simulink model "mass_spring_damper_AMPC_with_RLS"  (R2019b)
settings: Solver=VariableStepAuto  StartTime=0.0  StopTime=100  FixedStep=0.01  RelTol=1e-3
values from neighbouring files (symbols this model uses):
  A = AB(:,1:2)    [DMDc_MW.m]    (also in DMDc_param_sweep.m = real(A); EKF_msd_estimator.m = [0, 1; -k/m, -b/m]; HAVOK.m = AB(:,1:q*m); HAVOK_param_sweep.m = real(A))
  B = AB(:,end)    [DMDc_MW.m]    (also in DMDc_param_sweep.m = AB(:,(q*m+1):end); EKF_estimator.m = zeros(nx,1); EKF_msd_estimator.m = [0; 1/m]; HAVOK.m = AB(:,(q*m+1):end))
  C = [0 1]    [DMDc_MW.m]    (also in EKF_estimator.m = eye(6); EKF_msd_estimator.m = [1, 0]; KF_estimator.m = [1, 0]; LS.m)
  D = 0    [DMDc_MW.m]    (also in DMDc_param_sweep.m = (q-1)*Ts; EKF_estimator.m = m*L*L*(M+m*(1-Cx^2)); EKF_msd_estimator.m; HAVOK.m = 3.99)
  DX = [0; 0]    [DMDc_MW.m]    (also in LS.m; cart_pend_DMD_script.m; convert_model_for_AMPC.m; mass_spring_damper_DMD_script.m)
  nu = size_B(2)    [DMDc_MW.m]    (also in EKF_msd_estimator.m = 1; LS.m; Linear_regression_state_estimator.m = 2; cart_pend_DMD_script.m)
  ny = size_C(1)    [DMDc_MW.m]    (also in EKF_msd_estimator.m = 1; LS.m; Linear_regression_state_estimator.m = 1; cart_pend_DMD_script.m)
  p = 200    [HAVOK.m]    (also in cart_pend_HAVOK_N_train_time_sweep.m = p_saved(index); cart_pend_HAVOK_script.m = 40; floating_pend_2D_HAVOK_script.m = p_saved(save_index); mass_spring_damper_DMD_script.m = size(V)*[0; 1])
  U = zeros(nu,1)    [DMDc_MW.m]    (also in HAVOK.m = u_train(:, q:end-1); LS.m; Linear_regression_state_estimator.m = reshape(U, nx*nu,1); cart_pend_DMD_script.m)
  X = zeros(nx,1)    [DMDc_MW.m]    (also in LS.m; Linear_regression_parameter_estimator.m = [y_data(2:end-1)', y_data(1:end-2)', u_data(1:end-2)']; cart_pend_DMD_script.m; cart_pend_HAVOK_N_train_error_sweep.m = zeros(q*m,w))
  Y = zeros(ny,1)    [DMDc_MW.m]    (also in DMDc_param_sweep.m = zeros(q*m,w); HAVOK.m = zeros(q*m,w); HAVOK_param_sweep.m = zeros(q*m,w); LS.m)
undefined symbols (not defined in the file or in its folder): blk, iA, isLTV, lastPcov, lastu, lastx, MDscale, MVscale, nCC, nud, nv, nxp, nym, RMVscale, RYscale, ts, uoff, xoff, Yscale
libraries: mpcsigdimcheck_private x23
(part 1 of 2)
settings Model: Creator=Murray  LastModifiedBy=Murray

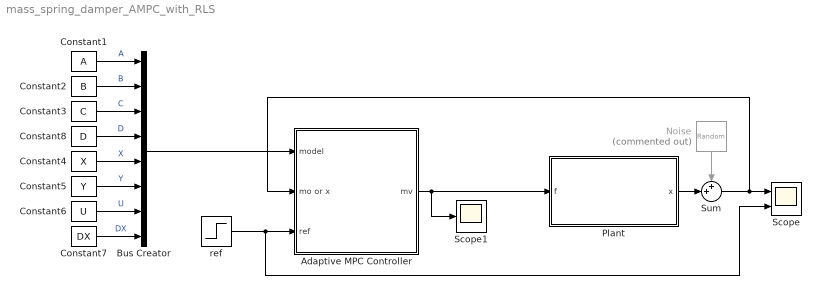
== system mass_spring_damper_AMPC_with_RLS ==
  Adaptive MPC Controller : Subsystem  AncestorBlock=mpclib/Adaptive MPC Controller  SCDEnableBlockLinearizationSpecification=on  InitFcn=ampcblock_InitFcn  StartFcn=ampcblock_StartFcn  mask(Adaptive MPC){mpcobj=mpc1, x0=, enable_value=0, updateMPCinCallerWorkspace=on, md_inport=off, mv_inport=off, uref_inport=off, return_cost=off, return_mvseq=off, return_qpstatus=off, return_xseq=off, return_state=off, return_ovseq=off, state_inport=off, isltv_plant=off, umin_inport=off, umax_inport=off, ymin_inport=off, ymax_inport=off, cc_inport=off, ywt_inport=off, uwt_inport=off, duwt_inport=off, rhoeps_inport=off, pm_inport=off, MaximumP=10, HorizonChoice=FixedHorizon, BlockDataType=double, SampleTimeInherited=off, switch_inport=off}
      mask prompts: mpcobj "MPC:general:BlgAMPC"; x0 "MPC:general:BlgState"; enable_value "Value enabling optimization"; updateMPCinCallerWorkspace "Update MPC object in caller workspace"; md_inport "MPC:general:BlgMD"; mv_inport "MPC:general:BlgEXTMV"; uref_inport "MPC:general:BlgMVTARGET"; return_cost "MPC:general:BlgCOST"; return_mvseq "MPC:general:BlgMVSEQ"; return_qpstatus "MPC:general:BlgQPSTATUS"; return_xseq "MPC:general:BlgXSEQ"; return_state "MPC:general:BlgESTSTATE"; return_ovseq "MPC:general:BlgOVSEQ"; state_inport "MPC:general:BlgXKK"; isltv_plant "MPC:general:BlgLTV"; umin_inport "MPC:general:BlgMVMin"; umax_inport "MPC:general:BlgMVMax"; ymin_inport "MPC:general:BlgOVMin"; ymax_inport "MPC:general:BlgOVMax"; cc_inport "Custom constraints (E, F, G, S)"; ywt_inport "MPC:general:BlgYWT"; uwt_inport "MPC:general:BlgUWT"; duwt_inport "MPC:general:BlgDUWT"; rhoeps_inport "MPC:general:BlgECRWT"; pm_inport "MPC:general:BlgPM"; MaximumP "MPC:general:BlgMaximumP"; HorizonChoice "Simulink:Variants:LabelComboBox"; BlockDataType "MPC:general:BlgDATATYPE"; SampleTimeInherited "MPC:general:BlgTS"; switch_inport "MPC:general:BlgSWITCH"
      mask help: MPC:utility:MaskDescAdaptiveMPC1
      mask init:
      | [blk,ts,A,B,C,D,isQP,strmoorx,nmoorx,nu,nv,ny,nx,nym,nud,...
      |     degrees,lastPcov,H,Hinv,Linv,iA,Ac,Kx,Ku1,Kut,Kr,Kv,...
      |     Mlim,Mx,Mu1,Mv,z_degrees,utarget,...
      |     lastx,lastu,p,xoff,uoff,yoff,voff,myoff,no_md,no_ref,...
      |     maxiter,CustomSolver,CustomSolverCodeGen,UseWarmStart,UseSuboptimalSolution,...
      |     nxQP,openloopflag,no_ym,no_mv,no_uref,...
      |     no_umin,no_umax,no_ymin,no_ymax,no_cc,...
      |     no_switch,CustomEstimation,...
      |     no_ywt, no_uwt, no_duwt, no_rhoeps,...
      |     Wy,Wdu,Jm,SuJm,Su1,Sx,Hv,Wu,I1,...
      |     isAdaptive, isLTV, Mrows, nCC, Ecc, Fcc, Scc, Gcc, Cid, Did, ...
      |     nxp, nup, nxid, mvindex, mdindex, unindex, myindex, ...
      |     Uscale, Yscale, MVscale, MDscale, ...
      |     RYscale,RMYscale,RMVscale,RMDscale,no_p,no_m,p0] = ampcblock_MaskInitFcnParameter();
      | ampcblock_MaskInitFcnResize(gcb,nv,nu,ny,nCC);
      mask Help: eval('mpcCSHelp(''MPCmaskAdaptive'',''HelpBrowser'')');
      mask Callback pm_inport: mpcblocks_callbackPM(gcb);
      mask TypeOptions HorizonChoice: MPC/optimizer/LabelModeActiveChoice
      mask DialogControl mpcobj Prompt: Adaptive MPC Controller
      mask DialogControl x0 Prompt: Initial Controller State
      mask DialogControl Container5 Prompt: MPC:general:BlgTab1
      mask DialogControl Container6 Prompt: MPC:general:BlgBox11
      mask DialogControl md_inport Prompt: Measured disturbance (md)
      mask DialogControl mv_inport Prompt: External manipulated variable (ext.mv)
      mask DialogControl uref_inport Prompt: Targets for manipulated variables (mv.target)
      mask DialogControl Container7 Prompt: MPC:general:BlgBox12
      mask DialogControl return_cost Prompt: Optimal cost (cost)
      mask DialogControl return_mvseq Prompt: Optimal control sequence (mv.seq)
      mask DialogControl return_qpstatus Prompt: Optimization status (qp.status)
      mask DialogControl return_xseq Prompt: Optimal state sequence (x.seq)
      mask DialogControl return_state Prompt: Estimated controller states (est.state)
      mask DialogControl return_ovseq Prompt: Optimal output sequence (y.seq)
      mask DialogControl Container16 Prompt: MPC:general:BlgBox13
      mask DialogControl state_inport Prompt: Use custom state estimation instead of using the built-in Kalman filter (x[k|k])
      mask DialogControl Container9 Prompt: MPC:general:BlgTab2
      mask DialogControl Container19 Prompt: MPC:general:BlgBox20
      mask DialogControl isltv_plant Prompt: Linear Time-Varying (LTV) plants (model expects 3-D signals)
      mask DialogControl Container10 Prompt: MPC:general:BlgBox21
      mask DialogControl umin_inport Prompt: Lower MV limits (umin)
      mask DialogControl umax_inport Prompt: Upper MV limits (umax)
      mask DialogControl ymin_inport Prompt: Lower OV limits (ymin)
      mask DialogControl ymax_inport Prompt: Upper OV limits (ymax)
      mask DialogControl Container11 Prompt: MPC:general:BlgBox22
      mask DialogControl ywt_inport Prompt: OV weights (y.wt)
      mask DialogControl uwt_inport Prompt: MV weights (u.wt)
      mask DialogControl duwt_inport Prompt: MVRate weights (du.wt)
      mask DialogControl rhoeps_inport Prompt: Slack variable weight (ecr.wt)
      mask DialogControl Container17 Prompt: Prediction and Control Horizons
      mask DialogControl pm_inport Prompt: Adjust prediction horizon (p) and control horizon (m) at run time
      mask DialogControl MaximumP Prompt: Maximum prediction horizon
      mask DialogControl HorizonChoice Prompt: Label mode active choice:
      mask DialogControl Container13 Prompt: MPC:general:BlgTab3
      mask DialogControl Container14 Prompt: MPC:general:BlgBox31
      mask DialogControl BlockDataType Prompt: Block Data Type
      mask DialogControl Container15 Prompt: MPC:general:BlgBox32
      mask DialogControl SampleTimeInherited Prompt: Inherit sample time (must be the same as controller sample time)
      mask DialogControl Container18 Prompt: MPC:general:BlgBox33
      mask DialogControl switch_inport Prompt: Use external signal to enable or disable optimization (switch)
      mask Display:
      | fprintf('Adaptive\nMPC');
      | port_label('output', 1, 'mv')
      | port_label('input', 1, 'model')
      | port_label('input', 2, 'mo')
      | port_label('input', 3, 'ref')
  Bus Creator : BusCreator  Inputs=A,B,C,D,X,Y,U,DX
  Constant1 : Constant  Value=A
  Constant2 : Constant  Value=B
  Constant3 : Constant  Value=C
  Constant4 : Constant  Value=X
  Constant5 : Constant  Value=Y
  Constant6 : Constant  Value=U
  Constant7 : Constant  Value=DX
  Constant8 : Constant  Value=D
  Noise : RandomNumber  Commented=on  Variance=0.00001  SampleTime=0.01
  Plant : Subsystem
  Scope : Scope  NumInputPorts=2
  Scope1 : Scope
  Sum : Sum  Inputs=++|
  ref : Step  SampleTime=0
  wires:
  ref/1 -> Adaptive MPC Controller/3(ref), Scope/2
  Adaptive MPC Controller/1(mv) -> Scope1/1, Plant/1(f)
  Constant1/1 -> Bus Creator/1  "A"
  Constant2/1 -> Bus Creator/2  "B"
  Constant6/1 -> Bus Creator/7  "U"
  Constant5/1 -> Bus Creator/6  "Y"
  Constant4/1 -> Bus Creator/5  "X"
  Constant8/1 -> Bus Creator/4  "D"
  Constant3/1 -> Bus Creator/3  "C"
  Bus Creator/1 -> Adaptive MPC Controller/1(model)
  Constant7/1 -> Bus Creator/8  "DX"
  Noise/1 -> Sum/1
  Plant/1(x) -> Sum/2
  Sum/1 -> Adaptive MPC Controller/2(mo or x), Scope/1

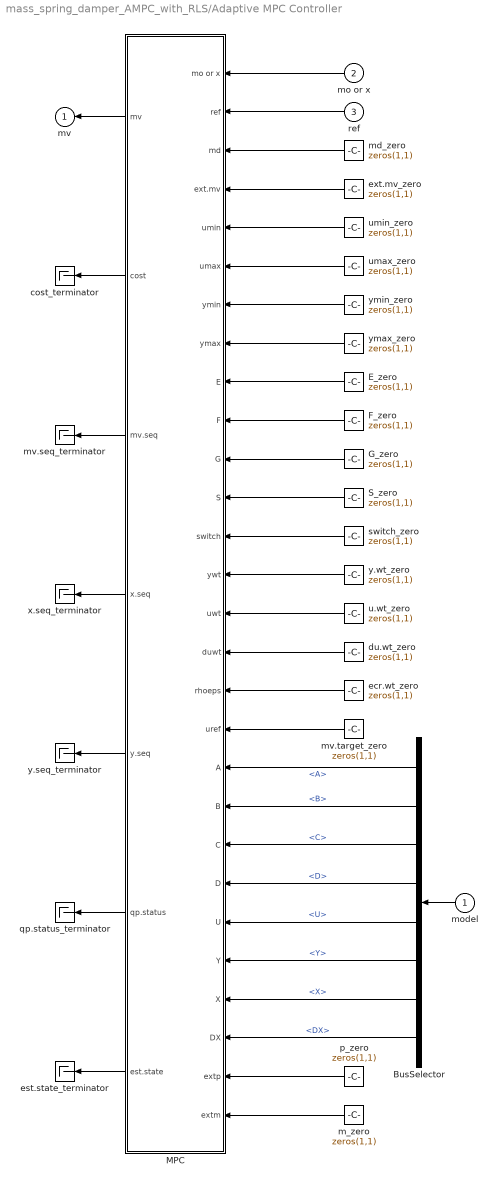
== system mass_spring_damper_AMPC_with_RLS/Adaptive MPC Controller ==
  model : Inport
  mo or x : Inport  Port=2
  ref : Inport  Port=3
  BusSelector : BusSelector  OutputSignals=A,B,C,D,U,Y,X,DX
  E_zero : Constant  Value=zeros(1,1)  VectorParams1D=off  OutDataTypeStr=BlockDataType
  F_zero : Constant  Value=zeros(1,1)  VectorParams1D=off  OutDataTypeStr=BlockDataType
  G_zero : Constant  Value=zeros(1,1)  VectorParams1D=off  OutDataTypeStr=BlockDataType
  MPC : Subsystem
  S_zero : Constant  Value=zeros(1,1)  VectorParams1D=off  OutDataTypeStr=BlockDataType
  cost_terminator : Terminator
  du.wt_zero : Constant  Value=zeros(1,1)  OutDataTypeStr=BlockDataType
  ecr.wt_zero : Constant  Value=zeros(1,1)  OutDataTypeStr=BlockDataType
  est.state_terminator : Terminator
  ext.mv_zero : Constant  Value=zeros(1,1)  OutDataTypeStr=BlockDataType
  m_zero : Constant  Value=zeros(1,1)  OutDataTypeStr=BlockDataType
  md_zero : Constant  Value=zeros(1,1)  OutDataTypeStr=BlockDataType
  mv.seq_terminator : Terminator
  mv.target_zero : Constant  Value=zeros(1,1)  OutDataTypeStr=BlockDataType
  p_zero : Constant  Value=zeros(1,1)  OutDataTypeStr=BlockDataType
  qp.status_terminator : Terminator
  switch_zero : Constant  Value=zeros(1,1)  OutDataTypeStr=BlockDataType
  u.wt_zero : Constant  Value=zeros(1,1)  OutDataTypeStr=BlockDataType
  umax_zero : Constant  Value=zeros(1,1)  OutDataTypeStr=BlockDataType
  umin_zero : Constant  Value=zeros(1,1)  OutDataTypeStr=BlockDataType
  x.seq_terminator : Terminator
  y.seq_terminator : Terminator
  y.wt_zero : Constant  Value=zeros(1,1)  OutDataTypeStr=BlockDataType
  ymax_zero : Constant  Value=zeros(1,1)  OutDataTypeStr=BlockDataType
  ymin_zero : Constant  Value=zeros(1,1)  OutDataTypeStr=BlockDataType
  mv : Outport  VectorParamsAs1DForOutWhenUnconnected=off
  wires:
  m_zero/1 -> MPC/28(extm)
  p_zero/1 -> MPC/27(extp)
  MPC/5(y.seq) -> y.seq_terminator/1
  MPC/4(x.seq) -> x.seq_terminator/1
  G_zero/1 -> MPC/11(G)
  F_zero/1 -> MPC/10(F)
  E_zero/1 -> MPC/9(E)
  S_zero/1 -> MPC/12(S)
  MPC/7(est.state) -> est.state_terminator/1
  y.wt_zero/1 -> MPC/14(ywt)
  switch_zero/1 -> MPC/13(switch)
  ymin_zero/1 -> MPC/7(ymin)
  umax_zero/1 -> MPC/6(umax)
  umin_zero/1 -> MPC/5(umin)
  u.wt_zero/1 -> MPC/15(uwt)
  ymax_zero/1 -> MPC/8(ymax)
  du.wt_zero/1 -> MPC/16(duwt)
  ecr.wt_zero/1 -> MPC/17(rhoeps)
  mv.target_zero/1 -> MPC/18(uref)
  ext.mv_zero/1 -> MPC/4(ext.mv)
  BusSelector/8 -> MPC/26(DX)  "<DX>"
  BusSelector/7 -> MPC/25(X)  "<X>"
  BusSelector/6 -> MPC/24(Y)  "<Y>"
  BusSelector/5 -> MPC/23(U)  "<U>"
  model/1 -> BusSelector/1
  BusSelector/4 -> MPC/22(D)  "<D>"
  BusSelector/3 -> MPC/21(C)  "<C>"
  BusSelector/2 -> MPC/20(B)  "<B>"
  BusSelector/1 -> MPC/19(A)  "<A>"
  MPC/6(qp.status) -> qp.status_terminator/1
  MPC/3(mv.seq) -> mv.seq_terminator/1
  MPC/2(cost) -> cost_terminator/1
  ref/1 -> MPC/2(ref)
  mo or x/1 -> MPC/1(mo or x)
  MPC/1(mv) -> mv/1
  md_zero/1 -> MPC/3(md)

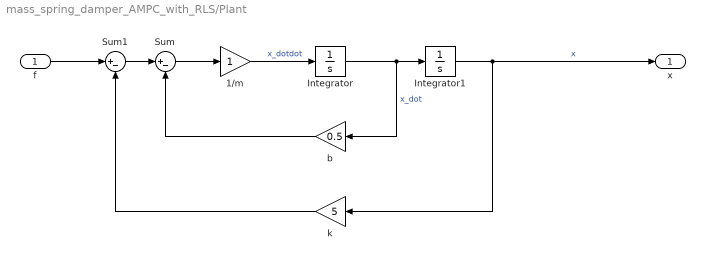
== system mass_spring_damper_AMPC_with_RLS/Plant ==
  f : Inport
  1/m : Gain
  Integrator : Integrator
  Integrator1 : Integrator
  Sum : Sum  Inputs=|+-
  Sum1 : Sum  Inputs=|+-
  b : Gain  Gain=0.5
  k : Gain  Gain=5
  x : Outport
  wires:
  f/1 -> Sum1/1
  Integrator/1 -> b/1, Integrator1/1  "x_dot"
  Sum1/1 -> Sum/1
  1/m/1 -> Integrator/1  "x_dotdot"
  Integrator1/1 -> x/1, k/1  "x"
  Sum/1 -> 1/m/1
  b/1 -> Sum/2
  k/1 -> Sum1/2

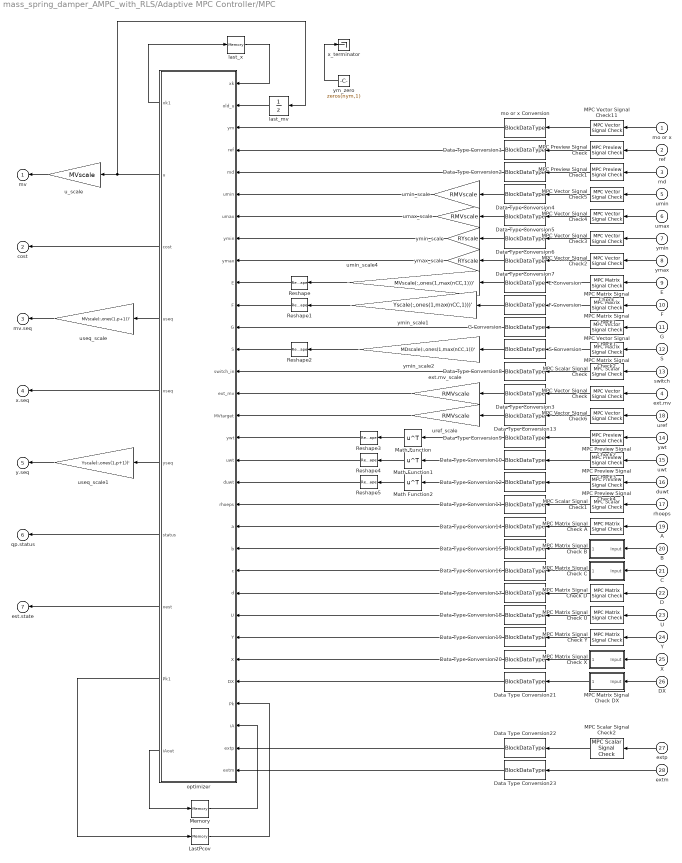
== system mass_spring_damper_AMPC_with_RLS/Adaptive MPC Controller/MPC ==
  mo or x : Inport
  ref : Inport  Port=2
  md : Inport  Port=3
  ext.mv : Inport  Port=4
  umin : Inport  Port=5
  umax : Inport  Port=6
  ymin : Inport  Port=7
  ymax : Inport  Port=8
  E : Inport  Port=9
  F : Inport  Port=10
  G : Inport  Port=11
  S : Inport  Port=12
  switch : Inport  Port=13
  ywt : Inport  Port=14
  uwt : Inport  Port=15
  duwt : Inport  Port=16
  rhoeps : Inport  Port=17
  uref : Inport  Port=18
  A : Inport  Port=19
  B : Inport  Port=20
  C : Inport  Port=21
  D : Inport  Port=22
  U : Inport  Port=23
  Y : Inport  Port=24
  X : Inport  Port=25
  DX : Inport  Port=26
  extp : Inport  Port=27
  extm : Inport  Port=28
  Data Type Conversion{1..23} (23 alike) : DataTypeConversion  OutDataTypeStr=BlockDataType
  E Conversion : DataTypeConversion  OutDataTypeStr=BlockDataType
  F Conversion : DataTypeConversion  OutDataTypeStr=BlockDataType
  G Conversion : DataTypeConversion  OutDataTypeStr=BlockDataType
  LastPcov : Memory  InitialCondition=lastPcov  InheritSampleTime=on  LinearizeAsDelay=on
  MPC Matrix Signal Check : mpcsigdimcheck_private/MPC Matrix Signal Check  blockname=blk  signalname='CustomConstraint.E'  numrow=max(nCC,1)  numcol=nu  steps=0  isLTV=0
      settings: SourceProductName=Model Predictive Control Toolbox  SourceProductBaseCode=MP
  MPC Matrix Signal Check A : mpcsigdimcheck_private/MPC Matrix Signal Check  blockname=blk  signalname='Model.A'  numrow=nxp  numcol=nxp  steps=p  isLTV=isLTV
      settings: SourceProductName=Model Predictive Control Toolbox  SourceProductBaseCode=MP
  MPC Matrix Signal Check B : Subsystem  AncestorBlock=mpcsigdimcheck_private/MPC Matrix Signal Check  mask(MPCSignalDimensionCheck){blockname=blk, signalname='Model.B', numrow=nxp, numcol=nu+nv-1+nud, steps=p, isLTV=isLTV}
      mask prompts: blockname "Block name"; signalname "Signal name"; numrow "Number of rows"; numcol "Number of columns"; steps "Number of prediction steps"; isLTV "Linear Time-Varying (LTV) plants"
      mask help: Internal use to check MPC input signal dimensions at compile time.
      mask init:
      | nrow = uint16(numrow);
      | ncol = uint16(numcol);
      | nsteps = uint16(steps);
      | isltv = uint16(isLTV);
  MPC Matrix Signal Check C : Subsystem  AncestorBlock=mpcsigdimcheck_private/MPC Matrix Signal Check  mask(MPCSignalDimensionCheck){blockname=blk, signalname='Model.C', numrow=ny, numcol=nxp, steps=p, isLTV=isLTV}
      mask prompts: blockname "Block name"; signalname "Signal name"; numrow "Number of rows"; numcol "Number of columns"; steps "Number of prediction steps"; isLTV "Linear Time-Varying (LTV) plants"
      mask help: Internal use to check MPC input signal dimensions at compile time.
      mask init:
      | nrow = uint16(numrow);
      | ncol = uint16(numcol);
      | nsteps = uint16(steps);
      | isltv = uint16(isLTV);
  MPC Matrix Signal Check D : mpcsigdimcheck_private/MPC Matrix Signal Check  blockname=blk  signalname='Model.D'  numrow=ny  numcol=nu+nv-1+nud  steps=p  isLTV=isLTV
      settings: SourceProductName=Model Predictive Control Toolbox  SourceProductBaseCode=MP
  MPC Matrix Signal Check DX : Subsystem  AncestorBlock=mpcsigdimcheck_private/MPC Matrix Signal Check  mask(MPCSignalDimensionCheck){blockname=blk, signalname='Model.DX', numrow=nxp, numcol=1, steps=p, isLTV=isLTV}
      mask prompts: blockname "Block name"; signalname "Signal name"; numrow "Number of rows"; numcol "Number of columns"; steps "Number of prediction steps"; isLTV "Linear Time-Varying (LTV) plants"
      mask help: Internal use to check MPC input signal dimensions at compile time.
      mask init:
      | nrow = uint16(numrow);
      | ncol = uint16(numcol);
      | nsteps = uint16(steps);
      | isltv = uint16(isLTV);
  MPC Matrix Signal Check U : mpcsigdimcheck_private/MPC Matrix Signal Check  blockname=blk  signalname='Model.U'  numrow=nu+nv-1+nud  numcol=1  steps=p  isLTV=isLTV
      settings: SourceProductName=Model Predictive Control Toolbox  SourceProductBaseCode=MP
  MPC Matrix Signal Check X : Subsystem  AncestorBlock=mpcsigdimcheck_private/MPC Matrix Signal Check  mask(MPCSignalDimensionCheck){blockname=blk, signalname='Model.X', numrow=nxp, numcol=1, steps=p, isLTV=isLTV}
      mask prompts: blockname "Block name"; signalname "Signal name"; numrow "Number of rows"; numcol "Number of columns"; steps "Number of prediction steps"; isLTV "Linear Time-Varying (LTV) plants"
      mask help: Internal use to check MPC input signal dimensions at compile time.
      mask init:
      | nrow = uint16(numrow);
      | ncol = uint16(numcol);
      | nsteps = uint16(steps);
      | isltv = uint16(isLTV);
  MPC Matrix Signal Check Y : mpcsigdimcheck_private/MPC Matrix Signal Check  blockname=blk  signalname='Model.Y'  numrow=ny  numcol=1  steps=p  isLTV=isLTV
      settings: SourceProductName=Model Predictive Control Toolbox  SourceProductBaseCode=MP
  MPC Matrix Signal Check1 : mpcsigdimcheck_private/MPC Matrix Signal Check  blockname=blk  signalname='CustomConstraint.F'  numrow=max(nCC,1)  numcol=ny  steps=0  isLTV=0
      settings: SourceProductName=Model Predictive Control Toolbox  SourceProductBaseCode=MP
  MPC Matrix Signal Check2 : mpcsigdimcheck_private/MPC Matrix Signal Check  blockname=blk  signalname='CustomConstraint.S'  numrow=max(nCC,1)  numcol=max(nv-1,1)  steps=0  isLTV=0
      settings: SourceProductName=Model Predictive Control Toolbox  SourceProductBaseCode=MP
  MPC Preview Signal Check : mpcsigdimcheck_private/MPC Preview Signal Check  blockname=blk  signalname='ref'  numrow=p  numcol=ny
      settings: SourceProductName=Model Predictive Control Toolbox  SourceProductBaseCode=MP
  MPC Preview Signal Check1 : mpcsigdimcheck_private/MPC Preview Signal Check  blockname=blk  signalname='md'  numrow=p+1  numcol=max(nv-1,1)
      settings: SourceProductName=Model Predictive Control Toolbox  SourceProductBaseCode=MP
  MPC Preview Signal Check2 : mpcsigdimcheck_private/MPC Preview Signal Check  blockname=blk  signalname='y.wt'  numrow=p  numcol=ny
      settings: SourceProductName=Model Predictive Control Toolbox  SourceProductBaseCode=MP
  MPC Preview Signal Check3 : mpcsigdimcheck_private/MPC Preview Signal Check  blockname=blk  signalname='u.wt'  numrow=p  numcol=nu
      settings: SourceProductName=Model Predictive Control Toolbox  SourceProductBaseCode=MP
  MPC Preview Signal Check4 : mpcsigdimcheck_private/MPC Preview Signal Check  blockname=blk  signalname='du.wt'  numrow=p  numcol=nu
      settings: SourceProductName=Model Predictive Control Toolbox  SourceProductBaseCode=MP
  MPC Scalar Signal Check : mpcsigdimcheck_private/MPC Scalar Signal Check  blockname=blk  signalname='switch'
      settings: SourceProductName=Model Predictive Control Toolbox  SourceProductBaseCode=MP
  MPC Scalar Signal Check1 : mpcsigdimcheck_private/MPC Scalar Signal Check  blockname=blk  signalname='ecr.wt'
      settings: SourceProductName=Model Predictive Control Toolbox  SourceProductBaseCode=MP
  MPC Scalar Signal Check2 : mpcsigdimcheck_private/MPC Scalar Signal Check  blockname=blk  signalname='p'
      settings: SourceProductName=Model Predictive Control Toolbox  SourceProductBaseCode=MP
  MPC Vector Signal Check : mpcsigdimcheck_private/MPC Vector Signal Check  blockname=blk  signalname='ext.mv'  num=nu  vectortype=Any
      settings: SourceProductName=Model Predictive Control Toolbox  SourceProductBaseCode=MP
  MPC Vector Signal Check1 : mpcsigdimcheck_private/MPC Vector Signal Check  blockname=blk  signalname='CustomConstraint.G'  num=max(nCC,1)  vectortype=Column
      settings: SourceProductName=Model Predictive Control Toolbox  SourceProductBaseCode=MP
  MPC Vector Signal Check11 : mpcsigdimcheck_private/MPC Vector Signal Check  blockname=blk  signalname=strmoorx  num=nmoorx  vectortype=Any
      settings: SourceProductName=Model Predictive Control Toolbox  SourceProductBaseCode=MP
  MPC Vector Signal Check2 : mpcsigdimcheck_private/MPC Vector Signal Check  blockname=blk  signalname='ymax'  num=ny  vectortype=Any
      settings: SourceProductName=Model Predictive Control Toolbox  SourceProductBaseCode=MP
  MPC Vector Signal Check3 : mpcsigdimcheck_private/MPC Vector Signal Check  blockname=blk  signalname='ymin'  num=ny  vectortype=Any
      settings: SourceProductName=Model Predictive Control Toolbox  SourceProductBaseCode=MP
  MPC Vector Signal Check4 : mpcsigdimcheck_private/MPC Vector Signal Check  blockname=blk  signalname='umax'  num=nu  vectortype=Any
      settings: SourceProductName=Model Predictive Control Toolbox  SourceProductBaseCode=MP
  MPC Vector Signal Check5 : mpcsigdimcheck_private/MPC Vector Signal Check  blockname=blk  signalname='umin'  num=nu  vectortype=Any
      settings: SourceProductName=Model Predictive Control Toolbox  SourceProductBaseCode=MP
  MPC Vector Signal Check6 : mpcsigdimcheck_private/MPC Vector Signal Check  blockname=blk  signalname='mv.target'  num=nu  vectortype=Any
      settings: SourceProductName=Model Predictive Control Toolbox  SourceProductBaseCode=MP
  Math Function : Math  Operator=transpose  SaturateOnIntegerOverflow=on
  Math Function1 : Math  Operator=transpose  SaturateOnIntegerOverflow=on
  Math Function2 : Math  Operator=transpose  SaturateOnIntegerOverflow=on
  Memory : Memory  InitialCondition=iA  InheritSampleTime=on  LinearizeAsDelay=on
  Reshape : Reshape  OutputDimensionality=Customize  OutputDimensions=double([max(nCC,1),nu])
  Reshape1 : Reshape  OutputDimensionality=Customize  OutputDimensions=double([max(nCC,1),ny])
  Reshape2 : Reshape  OutputDimensionality=Customize  OutputDimensions=double([max(nCC,1),max(nv-1,1)])
  Reshape3 : Reshape  OutputDimensionality=Column vector (2-D)
  Reshape4 : Reshape  OutputDimensionality=Column vector (2-D)
  Reshape5 : Reshape  OutputDimensionality=Column vector (2-D)
  S Conversion : DataTypeConversion  OutDataTypeStr=BlockDataType
  ext.mv_scale : Gain  Gain=RMVscale  SampleTime=ts
  last_mv : UnitDelay  InitialCondition=lastu+uoff  SampleTime=ts  HasFrameUpgradeWarning=on
  last_x : Memory  InitialCondition=lastx+xoff  InheritSampleTime=on  LinearizeAsDelay=on
  mo or x Conversion : DataTypeConversion  OutDataTypeStr=BlockDataType
  optimizer : Subsystem  VariantControlMode=Label  Variant=on  VariantControl=Variant1  LabelModeActiveChoice=FixedHorizon
  u_scale : Gain  Gain=MVscale  SampleTime=ts
  umax_scale : Gain  Gain=RMVscale  SampleTime=ts
  umin_scale : Gain  Gain=RMVscale  SampleTime=ts
  umin_scale4 : Gain  Gain=MVscale(:,ones(1,max(nCC,1)))'  SampleTime=ts
  uref_scale : Gain  Gain=RMVscale  SampleTime=ts
  useq_scale : Gain  Gain=MVscale(:,ones(1,p+1))'  SampleTime=ts
  useq_scale1 : Gain  Gain=Yscale(:,ones(1,p+1))'  SampleTime=ts
  x_terminator : Terminator
  ym_zero : Constant  Value=zeros(nym,1)  OutDataTypeStr=BlockDataType
  ymax_scale : Gain  Gain=RYscale  SampleTime=ts
  ymin_scale : Gain  Gain=RYscale  SampleTime=ts
  ymin_scale1 : Gain  Gain=Yscale(:,ones(1,max(nCC,1)))'  SampleTime=ts
  ymin_scale2 : Gain  Gain=MDscale(:,ones(1,max(nCC,1)))'  SampleTime=ts
  mv : Outport  OutDataTypeStr=BlockDataType  VectorParamsAs1DForOutWhenUnconnected=off
  cost : Outport  Port=2  OutDataTypeStr=BlockDataType  VectorParamsAs1DForOutWhenUnconnected=off
  mv.seq : Outport  Port=3  OutDataTypeStr=BlockDataType  VectorParamsAs1DForOutWhenUnconnected=off
  x.seq : Outport  Port=4  OutDataTypeStr=BlockDataType  VectorParamsAs1DForOutWhenUnconnected=off
  y.seq : Outport  Port=5  OutDataTypeStr=BlockDataType  VectorParamsAs1DForOutWhenUnconnected=off
  qp.status : Outport  Port=6  OutDataTypeStr=BlockDataType  VectorParamsAs1DForOutWhenUnconnected=off
  est.state : Outport  Port=7  OutDataTypeStr=BlockDataType  VectorParamsAs1DForOutWhenUnconnected=off
  wires:
  MPC Scalar Signal Check2/1 -> Data Type Conversion22/1
  extm/1 -> Data Type Conversion23/1
  extp/1 -> MPC Scalar Signal Check2/1
  Data Type Conversion23/1 -> optimizer/32(extm)
  Data Type Conversion22/1 -> optimizer/31(extp)
  optimizer/10(" iAout") -> Memory/1
  optimizer/9(" Pk1") -> LastPcov/1
  optimizer/8(" xest") -> est.state/1
  optimizer/7(" status") -> qp.status/1
  optimizer/6(" yseq") -> useq_scale1/1
  optimizer/5(" xseq") -> x.seq/1
  optimizer/4(" useq") -> useq_scale/1
  optimizer/3(" cost") -> cost/1
  optimizer/2(" u") -> last_mv/1, u_scale/1
  optimizer/1(" xk1") -> last_x/1
  Memory/1 -> optimizer/30("iA ")
  LastPcov/1 -> optimizer/29("Pk ")
  Data Type Conversion21/1 -> optimizer/28("DX ")
  Data Type Conversion20/1 -> optimizer/27("X ")
  Data Type Conversion19/1 -> optimizer/26("Y ")
  Data Type Conversion18/1 -> optimizer/25("U ")
  Data Type Conversion17/1 -> optimizer/24("d ")
  Data Type Conversion16/1 -> optimizer/23("c ")
  Data Type Conversion15/1 -> optimizer/22("b ")
  Data Type Conversion14/1 -> optimizer/21("a ")
  Data Type Conversion11/1 -> optimizer/20("rhoeps ")
  Reshape5/1 -> optimizer/19("duwt ")
  Reshape4/1 -> optimizer/18("uwt ")
  Reshape3/1 -> optimizer/17("ywt ")
  uref_scale/1 -> optimizer/16("MVtarget ")
  ext.mv_scale/1 -> optimizer/15("ext_mv ")
  Data Type Conversion8/1 -> optimizer/14("switch_in ")
  Reshape2/1 -> optimizer/13("S ")
  G Conversion/1 -> optimizer/12("G ")
  Reshape1/1 -> optimizer/11("F ")
  Reshape/1 -> optimizer/10("E ")
  ymax_scale/1 -> optimizer/9("ymax ")
  ymin_scale/1 -> optimizer/8("ymin ")
  umax_scale/1 -> optimizer/7("umax ")
  umin_scale/1 -> optimizer/6("umin ")
  Data Type Conversion2/1 -> optimizer/5("md ")
  Data Type Conversion1/1 -> optimizer/4("ref ")
  mo or x Conversion/1 -> optimizer/3("ym ")
  last_mv/1 -> optimizer/2("old_u ")
  last_x/1 -> optimizer/1("xk ")
  useq_scale1/1 -> y.seq/1
  Math Function2/1 -> Reshape5/1
  Math Function1/1 -> Reshape4/1
  Math Function/1 -> Reshape3/1
  MPC Matrix Signal Check1/1 -> F Conversion/1
  umin_scale4/1 -> Reshape/1
  ymin_scale1/1 -> Reshape1/1
  G/1 -> MPC Vector Signal Check1/1
  F/1 -> MPC Matrix Signal Check1/1
  E Conversion/1 -> umin_scale4/1
  ymin_scale2/1 -> Reshape2/1
  MPC Matrix Signal Check/1 -> E Conversion/1
  S/1 -> MPC Matrix Signal Check2/1
  E/1 -> MPC Matrix Signal Check/1
  MPC Matrix Signal Check2/1 -> S Conversion/1
  MPC Vector Signal Check1/1 -> G Conversion/1
  S Conversion/1 -> ymin_scale2/1
  F Conversion/1 -> ymin_scale1/1
  MPC Matrix Signal Check DX/1(Output) -> Data Type Conversion21/1
  MPC Matrix Signal Check X/1(Output) -> Data Type Conversion20/1
  MPC Matrix Signal Check Y/1 -> Data Type Conversion19/1
  MPC Matrix Signal Check U/1 -> Data Type Conversion18/1
  MPC Matrix Signal Check D/1 -> Data Type Conversion17/1
  MPC Matrix Signal Check C/1(Output) -> Data Type Conversion16/1
  MPC Matrix Signal Check B/1(Output) -> Data Type Conversion15/1
  MPC Matrix Signal Check A/1 -> Data Type Conversion14/1
  MPC Scalar Signal Check1/1 -> Data Type Conversion11/1
  MPC Preview Signal Check4/1 -> Data Type Conversion12/1
  MPC Preview Signal Check3/1 -> Data Type Conversion10/1
  MPC Preview Signal Check2/1 -> Data Type Conversion9/1
  MPC Vector Signal Check6/1 -> Data Type Conversion13/1
  MPC Vector Signal Check/1 -> Data Type Conversion3/1
  MPC Scalar Signal Check/1 -> Data Type Conversion8/1
  MPC Vector Signal Check2/1 -> Data Type Conversion7/1
  MPC Vector Signal Check3/1 -> Data Type Conversion6/1
  MPC Vector Signal Check4/1 -> Data Type Conversion5/1
  MPC Vector Signal Check5/1 -> Data Type Conversion4/1
  MPC Preview Signal Check1/1 -> Data Type Conversion2/1
  MPC Preview Signal Check/1 -> Data Type Conversion1/1
  MPC Vector Signal Check11/1 -> mo or x Conversion/1
  useq_scale/1 -> mv.seq/1
  u_scale/1 -> mv/1
  DX/1 -> MPC Matrix Signal Check DX/1(Input)
  X/1 -> MPC Matrix Signal Check X/1(Input)
  Y/1 -> MPC Matrix Signal Check Y/1
  U/1 -> MPC Matrix Signal Check U/1
  D/1 -> MPC Matrix Signal Check D/1
  C/1 -> MPC Matrix Signal Check C/1(Input)
  B/1 -> MPC Matrix Signal Check B/1(Input)
  A/1 -> MPC Matrix Signal Check A/1
  md/1 -> MPC Preview Signal Check1/1
  umin/1 -> MPC Vector Signal Check5/1
  umax/1 -> MPC Vector Signal Check4/1
  ymin/1 -> MPC Vector Signal Check3/1
  ymax/1 -> MPC Vector Signal Check2/1
  switch/1 -> MPC Scalar Signal Check/1
  ext.mv/1 -> MPC Vector Signal Check/1
  Data Type Conversion3/1 -> ext.mv_scale/1
  ref/1 -> MPC Preview Signal Check/1
  mo or x/1 -> MPC Vector Signal Check11/1
  ywt/1 -> MPC Preview Signal Check2/1
  uwt/1 -> MPC Preview Signal Check3/1
  Data Type Conversion4/1 -> umin_scale/1
  Data Type Conversion5/1 -> umax_scale/1
  Data Type Conversion7/1 -> ymax_scale/1
  Data Type Conversion9/1 -> Math Function/1
  Data Type Conversion12/1 -> Math Function2/1
  Data Type Conversion6/1 -> ymin_scale/1
  rhoeps/1 -> MPC Scalar Signal Check1/1
  duwt/1 -> MPC Preview Signal Check4/1
  Data Type Conversion10/1 -> Math Function1/1
  uref/1 -> MPC Vector Signal Check6/1
  Data Type Conversion13/1 -> uref_scale/1
  ym_zero/1 -> x_terminator/1

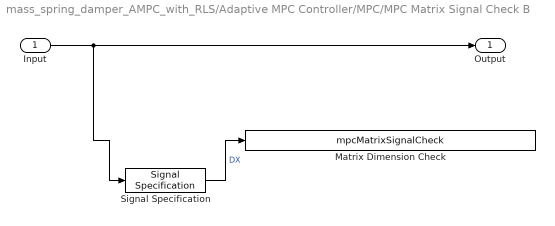
== system mass_spring_damper_AMPC_with_RLS/Adaptive MPC Controller/MPC/MPC Matrix Signal Check B ==
  Input : Inport
  Matrix Dimension Check : S-Function  FunctionName=mpcMatrixSignalCheck  Parameters=blockname, signalname, nrow, ncol, nsteps, isltv  SFunctionDeploymentMode=off  EnableBusSupport=off
  Signal Specification : SignalSpecification  Dimensions=[2 1]
  Output : Outport  VectorParamsAs1DForOutWhenUnconnected=off
  wires:
  Input/1 -> Output/1, Signal Specification/1
  Signal Specification/1 -> Matrix Dimension Check/1  "DX"

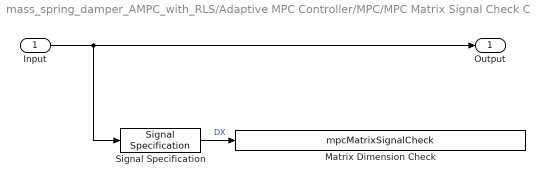
== system mass_spring_damper_AMPC_with_RLS/Adaptive MPC Controller/MPC/MPC Matrix Signal Check C ==
  Input : Inport
  Matrix Dimension Check : S-Function  FunctionName=mpcMatrixSignalCheck  Parameters=blockname, signalname, nrow, ncol, nsteps, isltv  SFunctionDeploymentMode=off  EnableBusSupport=off
  "Signal Specification " : SignalSpecification  Dimensions=[1 2]
  Output : Outport  VectorParamsAs1DForOutWhenUnconnected=off
  wires:
  Input/1 -> Output/1, "Signal Specification "/1
  "Signal Specification "/1 -> Matrix Dimension Check/1  "DX"

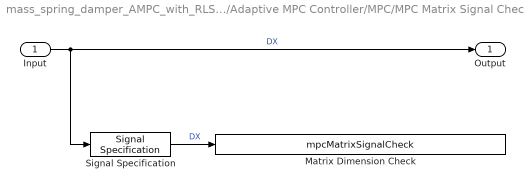
== system mass_spring_damper_AMPC_with_RLS/Adaptive MPC Controller/MPC/MPC Matrix Signal Check DX ==
  Input : Inport
  Matrix Dimension Check : S-Function  FunctionName=mpcMatrixSignalCheck  Parameters=blockname, signalname, nrow, ncol, nsteps, isltv  SFunctionDeploymentMode=off  EnableBusSupport=off
  Signal Specification : SignalSpecification  Dimensions=[2 1]
  Output : Outport  VectorParamsAs1DForOutWhenUnconnected=off
  wires:
  Input/1 -> Signal Specification/1, Output/1  "DX"
  Signal Specification/1 -> Matrix Dimension Check/1  "DX"

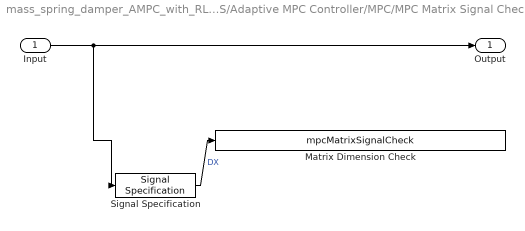
== system mass_spring_damper_AMPC_with_RLS/Adaptive MPC Controller/MPC/MPC Matrix Signal Check X ==
  Input : Inport
  Matrix Dimension Check : S-Function  FunctionName=mpcMatrixSignalCheck  Parameters=blockname, signalname, nrow, ncol, nsteps, isltv  SFunctionDeploymentMode=off  EnableBusSupport=off
  Signal Specification : SignalSpecification  Dimensions=[2 1]
  Output : Outport  VectorParamsAs1DForOutWhenUnconnected=off
  wires:
  Input/1 -> Output/1, Signal Specification/1
  Signal Specification/1 -> Matrix Dimension Check/1  "DX"

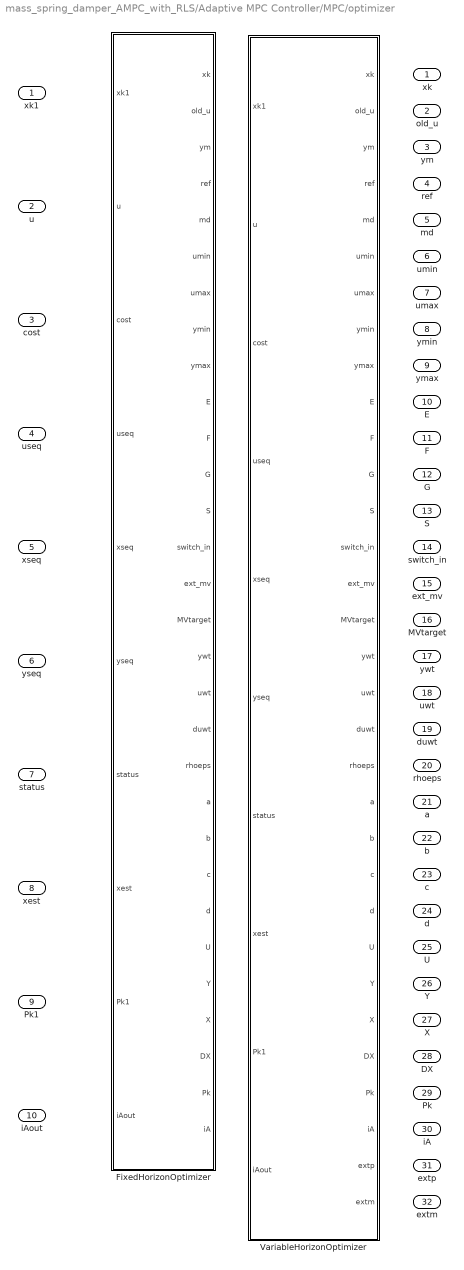
== system mass_spring_damper_AMPC_with_RLS/Adaptive MPC Controller/MPC/optimizer ==
  "xk " : Inport
  "old_u " : Inport  Port=2
  "ym " : Inport  Port=3
  "ref " : Inport  Port=4
  "md " : Inport  Port=5
  "umin " : Inport  Port=6
  "umax " : Inport  Port=7
  "ymin " : Inport  Port=8
  "ymax " : Inport  Port=9
  "E " : Inport  Port=10
  "F " : Inport  Port=11
  "G " : Inport  Port=12
  "S " : Inport  Port=13
  "switch_in " : Inport  Port=14
  "ext_mv " : Inport  Port=15
  "MVtarget " : Inport  Port=16
  "ywt " : Inport  Port=17
  "uwt " : Inport  Port=18
  "duwt " : Inport  Port=19
  "rhoeps " : Inport  Port=20
  "a " : Inport  Port=21
  "b " : Inport  Port=22
  "c " : Inport  Port=23
  "d " : Inport  Port=24
  "U " : Inport  Port=25
  "Y " : Inport  Port=26
  "X " : Inport  Port=27
  "DX " : Inport  Port=28
  "Pk " : Inport  Port=29
  "iA " : Inport  Port=30
  extp : Inport  Port=31
  extm : Inport  Port=32
  FixedHorizonOptimizer : MATLAB Function  VariantControl=FixedHorizon
  VariableHorizonOptimizer : MATLAB Function  VariantControl=VariableHorizon
  " xk1" : Outport  VectorParamsAs1DForOutWhenUnconnected=off
  " u" : Outport  Port=2  VectorParamsAs1DForOutWhenUnconnected=off
  " cost" : Outport  Port=3  VectorParamsAs1DForOutWhenUnconnected=off
  " useq" : Outport  Port=4  VectorParamsAs1DForOutWhenUnconnected=off
  " xseq" : Outport  Port=5  VectorParamsAs1DForOutWhenUnconnected=off
  " yseq" : Outport  Port=6  VectorParamsAs1DForOutWhenUnconnected=off
  " status" : Outport  Port=7  VectorParamsAs1DForOutWhenUnconnected=off
  " xest" : Outport  Port=8  VectorParamsAs1DForOutWhenUnconnected=off
  " Pk1" : Outport  Port=9  VectorParamsAs1DForOutWhenUnconnected=off
  " iAout" : Outport  Port=10  VectorParamsAs1DForOutWhenUnconnected=off

== matlab function mass_spring_damper_AMPC_with_RLS/Adaptive MPC Controller/MPC/optimizer/FixedHorizonOptimizer ==
  settings: updateMethod=DISCRETE  sampleTime=ts
  data: xk1 output BlockDataType; xk input BlockDataType; old_u input BlockDataType; ym input BlockDataType; ref input BlockDataType; md input BlockDataType; umin input BlockDataType; umax input BlockDataType; ymin input BlockDataType; ymax input BlockDataType; E input BlockDataType; F input BlockDataType; G input BlockDataType; S input BlockDataType; switch_in input BlockDataType; ext_mv input BlockDataType; MVtarget input BlockDataType; isQP parameter boolean; nx parameter BlockDataType; nxp parameter BlockDataType; nup parameter BlockDataType; nu parameter BlockDataType; ny parameter BlockDataType; degrees parameter BlockDataType; Hinv parameter BlockDataType; Kx parameter BlockDataType; Ku1 parameter BlockDataType; Kut parameter BlockDataType; Kr parameter BlockDataType; Kv parameter BlockDataType; Mlim parameter BlockDataType; Mx parameter BlockDataType; Mu1 parameter BlockDataType; Mv parameter BlockDataType; z_degrees parameter BlockDataType; utarget parameter BlockDataType; p parameter BlockDataType; maxiter parameter BlockDataType; CustomSolver parameter boolean; CustomSolverCodeGen parameter boolean; UseWarmStart parameter boolean; UseSuboptimalSolution parameter boolean; nxQP parameter BlockDataType; openloopflag parameter boolean; no_umin parameter BlockDataType; no_umax parameter BlockDataType; no_ymin parameter BlockDataType; no_ymax parameter BlockDataType; switch_inport parameter BlockDataType; no_switch parameter BlockDataType; enable_value parameter BlockDataType; return_cost parameter BlockDataType; H parameter BlockDataType; return_mvseq parameter BlockDataType; return_xseq parameter BlockDataType; return_ovseq parameter BlockDataType; Linv parameter BlockDataType; Ac parameter BlockDataType; ywt input BlockDataType; uwt input BlockDataType; duwt input BlockDataType; rhoeps input BlockDataType; isLTV parameter boolean; a input BlockDataType; b input BlockDataType; c input BlockDataType; d input BlockDataType; U input BlockDataType; Y input BlockDataType; X input BlockDataType; DX input BlockDataType; Pk input BlockDataType; iA input boolean; u output BlockDataType; cost output BlockDataType; useq output BlockDataType; xseq output BlockDataType; yseq output BlockDataType; status output BlockDataType; xest output BlockDataType; Pk1 output BlockDataType; no_ywt parameter BlockDataType; no_uwt parameter BlockDataType; no_duwt parameter BlockDataType; no_rhoeps parameter BlockDataType; Wy parameter BlockDataType; Wdu parameter BlockDataType; Jm parameter BlockDataType; SuJm parameter BlockDataType; Su1 parameter BlockDataType; Sx parameter BlockDataType; Hv parameter BlockDataType; Wu parameter BlockDataType; I1 parameter BlockDataType; iAout output boolean; A parameter BlockDataType; C parameter BlockDataType; B parameter BlockDataType; D parameter BlockDataType; Cid parameter BlockDataType; Did parameter BlockDataType; Mrows parameter BlockDataType; nCC parameter BlockDataType; Ecc parameter BlockDataType; Fcc parameter BlockDataType; Scc parameter BlockDataType; Gcc parameter BlockDataType; nv parameter BlockDataType; no_md parameter BlockDataType; no_ref parameter BlockDataType; no_uref parameter BlockDataType; no_mv parameter BlockDataType; RYscale parameter BlockDataType; RMDscale parameter BlockDataType; myindex parameter BlockDataType; xoff parameter BlockDataType; CustomEstimation parameter boolean; mvindex parameter BlockDataType; mdindex parameter BlockDataType; unindex parameter BlockDataType; nxid parameter BlockDataType; Uscale parameter BlockDataType; Yscale parameter BlockDataType; uoff parameter BlockDataType; voff parameter BlockDataType; yoff parameter BlockDataType; myoff parameter BlockDataType; no_cc parameter BlockDataType
function [xk1, u, cost, useq, xseq, yseq, status, xest, Pk1, iAout] = fcn(...
            xk, old_u, ym, ref, md, umin, umax, ymin, ymax, E, F, G, S,...
            switch_in, ext_mv, MVtarget, isQP, nx, nxp, nup, ...
            nu, ny, degrees, Hinv, Kx, Ku1, Kut, Kr, Kv, Mlim, ...
            Mx, Mu1, Mv, z_degrees, utarget, p, maxiter, ...
            CustomSolver, CustomSolverCodeGen, UseWarmStart, UseSuboptimalSolution, nxQP, openloopflag, ...
            no_umin, no_umax, no_ymin, no_ymax, switch_inport, no_switch, enable_value, ...
            return_cost, H, return_mvseq, return_xseq, return_ovseq, Linv, Ac, ...
            ywt, uwt, duwt, rhoeps, isLTV, a, b, c, d, U, Y, X, DX, Pk, iA, ...
            no_ywt, no_uwt, no_duwt, no_rhoeps,...
            Wy, Wdu, Jm, SuJm, Su1, Sx, Hv, Wu, I1, ...
            A, C, B, D, Cid, Did, Mrows, nCC, Ecc, Fcc, Scc, Gcc, ...
            nv, no_md, no_ref, no_uref, no_mv, RYscale, RMDscale, myindex, ...
            xoff, CustomEstimation, mvindex, mdindex, unindex, nxid, Uscale, Yscale, uoff, voff, yoff, myoff, no_cc)
%#codegen
coder.extrinsic('mpcblock_optimizer_double_mex');
coder.extrinsic('mpcblock_optimizer_single_mex');
coder.extrinsic('mpcblock_refmd_double_mex');
coder.extrinsic('mpcblock_refmd_single_mex');

% Constants
isSimulation = coder.target('Sfun') && ~coder.target('RtwForRapid') && ~coder.target('RtwForSim');
isAdaptive = ~isLTV; % isLTV=true forces isAdaptive=false
isDouble = isa(ref,'double');
if isDouble
    DataType = 'double';
else
    DataType = 'single';
end
ZERO = zeros('like',ref);
ONE = ones('like',ref);
hasMD = nv>1;

% Pre-allocate all the MEX block outputs for the simulation mode
%#ok<*NASGU>
if isSimulation
    rseq = zeros(p*ny,1,'like',ref); %#ok<*NASGU>
    vseq = zeros((p+1)*nv,1,'like',ref);
    v = zeros(nv,1,'like',ref);
    xk1 = zeros(nx,1,'like',ref);
    u = zeros(nu,1,'like',ref);
    cost = ZERO;
    useq = zeros(p+1,nu,'like',ref); %#ok<*PREALL>
    status = ONE;
    xest = zeros(nx,1,'like',ref);
    iAout = iA;
end

% Model update
nym = length(myindex);
ai=zeros(nxp,nxp,'like',ref);
bi=zeros(nxp,nup,'like',ref);
ci=zeros(ny,nxp,'like',ref);
di=zeros(ny,nup,'like',ref);

ai(:,:)=a(:,:,1);
bi(:,:)=b(:,:,1);
ci(:,:)=c(:,:,1);
di(:,:)=d(:,:,1);

% Allocate matrices. Must allocate 3D matrix also in Adaptive case,
% otherwise EML code does not compile.
Bu=zeros(nx,nu,p+1,'like',ref);
Bv=zeros(nx,nv,p+1,'like',ref);
Dv=zeros(ny,nv,p+1,'like',ref);
Dvm=zeros(nym,nv,p+1,'like',ref);
Cm=zeros(nym,nx,p+1,'like',ref);
if ~isLTV
    % Adaptive
    [A(:,:,1),C(:,:,1),Bu(:,:,1),Bv(:,:,1),Cm(:,:,1),Dv(:,:,1),Dvm(:,:,1),Qk,Rk,Nk] = mpc_plantupdate(...
        ai,bi,ci,di,A(:,:,1),B(:,:,1),C(:,:,1),D(:,:,1),mvindex,mdindex,unindex,nxp,nup,ny,nv,nxid, ...
        myindex,Uscale,Yscale,Cid,Did);
else
    % Retrieve LTV model
    for i=1:p+1
        ai(1:nxp,1:nxp)=a(:,:,i);
        bi(1:nxp,1:nup)=b(:,:,i);
        ci(1:ny,1:nxp)=c(:,:,i);
        di(1:ny,1:nup)=d(:,:,i);
        [A(:,:,i),C(:,:,i),Bu(:,:,i),Bv(:,:,i),Cm(:,:,i),Dv(:,:,i),Dvm(:,:,i),Qk,Rk,Nk] =...
            mpc_plantupdate(ai,bi,ci,di,A(:,:,i),B(:,:,i),C(:,:,i),D(:,:,i),mvindex,mdindex,unindex,nxp,nup,ny,nv,nxid, ...
            myindex,Uscale,Yscale,Cid,Did);
    end
end

% Offset update together with Mlim, utarget, Bv and Dv values
[Mlim, utarget, uoff, voff, yoff, myoff, xoff, Bv, Dv] = ...
    mpc_updateFromNominal(isAdaptive,isQP,p,Mlim,Mrows,...
       U,Uscale,uoff,mvindex,voff,mdindex,utarget,nu,nv-1,...
       Y,Yscale,yoff,myoff,myindex,ny,...
       X,xoff,nxp,DX,A,Bu,Bv,C,Dv,nCC);

% Remove last u offset
old_u = old_u - uoff;       

% Get reference and MD signals -- accounting for previewing
if isSimulation
    if isDouble
        [rseq, vseq, v] = mpcblock_refmd_double_mex(ref,md,nv,ny,p,yoff,voff,no_md,no_ref,openloopflag, RYscale, RMDscale);
    else
        [rseq, vseq, v] = mpcblock_refmd_single_mex(ref,md,nv,ny,p,yoff,voff,no_md,no_ref,openloopflag, RYscale, RMDscale);        
    end
else
    % When doing code generation, use M code directly
    [rseq, vseq, v] = mpcblock_refmd(ref,md,nv,ny,p,yoff,voff,no_md,no_ref,openloopflag, RYscale, RMDscale);
end

% External MV override.  
% NOTE: old_u and ext_mv input signals are dimensionless and offset-free.
if no_mv==ONE
    % no external mv: old_u is the optimal u[k-1] from last_mv
    delmv = zeros(nu,1,'like',ref);
else
    % has external mv: old_u is the external u[k-1]
    ext_mv = ext_mv - uoff;     % bias correction
    delmv = ext_mv - old_u;
    old_u = ext_mv;
end

% Obtain x[k|k]
xk = xk - xoff;     % Remove offset
if CustomEstimation==ONE
    % Input is x(k|k)
    xest = xk;
else
    % Calculate gain matrices, and perform measurement update.
    Kinv = eye(nym,'like',ref)/(Cm(:,:,1)*Pk*Cm(:,:,1)' + Rk);
    L = (A(:,:,1)*Pk*Cm(:,:,1)' + Nk)*Kinv;
    M = Pk*Cm(:,:,1)'*Kinv;
    % LTVKF state estimation.
    % Scale measured output and remove offset.
    ym = ym.*RYscale(myindex) - myoff;
    % Correct x(k|k-1) for possible external mv override.
    % NOTE:  Offset was removed from x[k|k-1] at k=0.
    xk = xk + Bu(:,:,1)*delmv;
    % Measurement upate to x(k|k)
    ym_est = Cm(:,:,1)*xk + Dvm(:,:,1)*v;
    y_innov = ym - ym_est;
    xest = xk + M*y_innov;
end

% Real-time MV target override
% Note: utargetValue is a vector length p*nu.  
if no_uref==ONE
    % no external utarget
    utargetValue = utarget;
else
    % Define constant targets for the entire horizon.
    MVtarget = MVtarget - uoff;         % Bias correction
    utargetValue = reshape(MVtarget(:,ones(p,1)),nu*p,1);
end

% Real-time custom constraint override (scaled E/F/S)
if no_cc~=ONE
    Ecc = E;
    Fcc = F;
    Gcc = G;
    if nv>1
        Scc = S;
    end
end

return_sequence = (return_mvseq || return_xseq || return_ovseq)*ONE;
if isSimulation
    if isDouble
        [u, cost, useq, status, iAout] = mpcblock_optimizer_double_mex(...
            rseq, vseq, umin, umax, ymin, ymax, switch_in, xest, old_u, iA, ...
            isQP, nu, ny, degrees, Hinv, Kx, Ku1, Kut, Kr, Kv, Mlim, ...
            Mx, Mu1, Mv, z_degrees, utargetValue, p, uoff, voff, yoff, maxiter, ...
            CustomSolver, false, UseWarmStart, UseSuboptimalSolution, nxQP, openloopflag, ...
            no_umin, no_umax, no_ymin, no_ymax, no_cc, switch_inport, ...
            no_switch, enable_value, return_cost, H, return_sequence, Linv, Ac, ...
            ywt, uwt, duwt, rhoeps, no_ywt, no_uwt, no_duwt, no_rhoeps,...
            Wy, Wdu, Jm, SuJm, Su1, Sx, Hv, Wu, I1, ...
            isAdaptive, isLTV, A, Bu, Bv, C, Dv, ...
            Mrows, nCC, Ecc, Fcc, Scc, Gcc);    
    else
        [u, cost, useq, status, iAout] = mpcblock_optimizer_single_mex(...
            rseq, vseq, umin, umax, ymin, ymax, switch_in, xest, old_u, iA, ...
            isQP, nu, ny, degrees, Hinv, Kx, Ku1, Kut, Kr, Kv, Mlim, ...
            Mx, Mu1, Mv, z_degrees, utargetValue, p, uoff, voff, yoff, maxiter, ...
            CustomSolver, false, UseWarmStart, UseSuboptimalSolution, nxQP, openloopflag, ...
            no_umin, no_umax, no_ymin, no_ymax, no_cc, switch_inport, ...
            no_switch, enable_value, return_cost, H, return_sequence, Linv, Ac, ...
            ywt, uwt, duwt, rhoeps, no_ywt, no_uwt, no_duwt, no_rhoeps,...
            Wy, Wdu, Jm, SuJm, Su1, Sx, Hv, Wu, I1, ...
            isAdaptive, isLTV, A, Bu, Bv, C, Dv, ...
            Mrows, nCC, Ecc, Fcc, Scc, Gcc);    
    end
else
    % When doing code generation, use M code directly
        [u, cost, useq, status, iAout] = mpcblock_optimizer(...
            rseq, vseq, umin, umax, ymin, ymax, switch_in, xest, old_u, iA, ...
            isQP, nu, ny, degrees, Hinv, Kx, Ku1, Kut, Kr, Kv, Mlim, ...
            Mx, Mu1, Mv, z_degrees, utargetValue, p, uoff, voff, yoff, maxiter, ...
            false, CustomSolverCodeGen, UseWarmStart, UseSuboptimalSolution, nxQP, openloopflag, ...
            no_umin, no_umax, no_ymin, no_ymax, no_cc, switch_inport, ...
            no_switch, enable_value, return_cost, H, return_sequence, Linv, Ac, ...
            ywt, uwt, duwt, rhoeps, no_ywt, no_uwt, no_duwt, no_rhoeps,...
            Wy, Wdu, Jm, SuJm, Su1, Sx, Hv, Wu, I1, ...
            isAdaptive, isLTV, A, Bu, Bv, C, Dv, ...
            Mrows, nCC, Ecc, Fcc, Scc, Gcc);    
end

if return_xseq || return_ovseq
    [yseq, xseq] = mpc_computeSequence(isLTV, xest, useq, vseq, uoff, yoff, xoff, p, ny, nxQP, nv, A, Bu, Bv, C, Dv);
else
    yseq = zeros(p+1,ny,'like',rseq);
    xseq = zeros(p+1,nxQP,'like',rseq);
end

if CustomEstimation==ONE
    xk1 = zeros(nx,1,'like',ref);
    Pk1 = Pk;
else
    % LTVKF state and covariance update
    xk1 = A(:,:,1)*xk + Bu(:,:,1)*(u - uoff) + Bv(:,:,1)*v + L*y_innov;
    Pk1 = A(:,:,1)*Pk*A(:,:,1)' - (A(:,:,1)*Pk*Cm(:,:,1)' + Nk)*L' + Qk;
    Pk1 = 0.5*(Pk1 + Pk1'); % guarantee symmetric for numerical stability
end
xk1 = xk1 + xoff;   % Updated state must include offset

% return xest in original value
xest = xest + xoff;
